simulink model "DroneControl"  (R2016a)
settings: Solver=VariableStepAuto  StartTime=0.0  StopTime=20  RelTol=1e-3
values from neighbouring files (symbols this model uses):
  SetPoint = 50    [DroneScript.m]
libraries: simulink x1
settings Model: Creator=Radu  LastModifiedBy=Radu

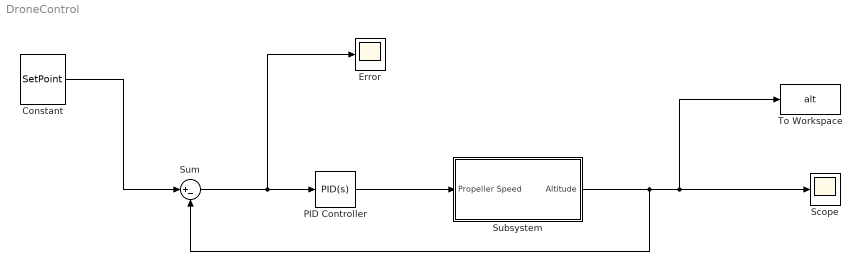
== system DroneControl ==
  Constant : Constant  Value=SetPoint
  "Error " : Scope
  PID Controller : simulink/Continuous/PID Controller  Controller=PID  TimeDomain=Continuous-time  SampleTime=-1  IntegratorMethod=Forward Euler  FilterMethod=Forward Euler  Form=Parallel  UseFilter=on  ControllerParametersSource=internal  P=10  I=1  D=0.1  N=100  InitialConditionSource=internal  InitialConditionForIntegrator=0  InitialConditionForFilter=0  ExternalReset=none  LimitOutput=off  UpperSaturationLimit=inf  LowerSaturationLimit=-inf  LinearizeAsGain=on  AntiWindupMode=none  Kb=1  TrackingMode=off  Kt=1  PParamMin=[]  PParamMax=[]  IParamMin=[]  IParamMax=[]  DParamMin=[]  DParamMax=[]  NParamMin=[]  NParamMax=[]  KbParamMin=[]  KbParamMax=[]  KtParamMin=[]  KtParamMax=[]  POutMin=[]  POutMax=[]  IOutMin=[]  IOutMax=[]  DOutMin=[]  DOutMax=[]  NOutMin=[]  NOutMax=[]  KbOutMin=[]  KbOutMax=[]  KtOutMin=[]  KtOutMax=[]  IntegratorOutMin=[]  IntegratorOutMax=[]  FilterOutMin=[]  FilterOutMax=[]  SumOutMin=[]  SumOutMax=[]  SumI1OutMin=[]  SumI1OutMax=[]  SumI2OutMin=[]  SumI2OutMax=[]  SumI3OutMin=[]  SumI3OutMax=[]  SumDOutMin=[]  SumDOutMax=[]  SaturationOutMin=[]  SaturationOutMax=[]  IntegratorContinuousStateAttributes=''  IntegratorStateMustResolveToSignalObject=off  IntegratorRTWStateStorageClass=Auto  FilterContinuousStateAttributes=''  FilterStateMustResolveToSignalObject=off  FilterRTWStateStorageClass=Auto  DifferentiatorICPrevScaledInput=0  DifferentiatorOutMin=[]  DifferentiatorOutMax=[]
  Scope : Scope
  Subsystem : Subsystem
  Sum : Sum  Inputs=|+-
  To Workspace : ToWorkspace  VariableName=alt  SaveFormat=Timeseries  SampleTime=-1
  wires:
  Subsystem/1(Altitude) -> To Workspace/1, Scope/1, Sum/2
  PID Controller/1 -> Subsystem/1(Propeller Speed)
  Sum/1 -> "Error "/1, PID Controller/1
  Constant/1 -> Sum/1

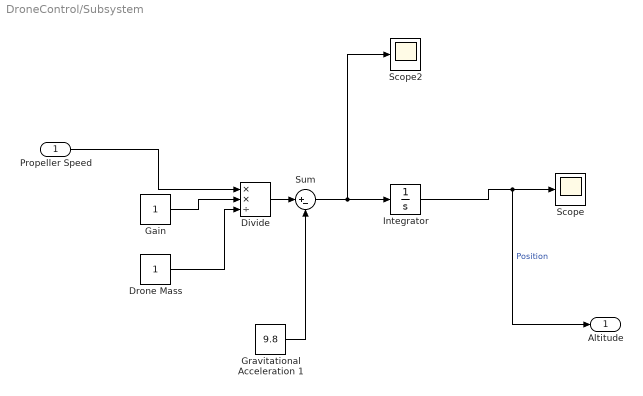
== system DroneControl/Subsystem ==
  Propeller Speed : Inport
  Divide : Product  Inputs=**/
  "Drone Mass " : Constant
  "Gain " : Constant
  Gravitational Acceleration 1 : Constant  Value=9.8
  Integrator : Integrator  LimitOutput=on  LowerSaturationLimit=0
  Scope : Scope
  Scope2 : Scope
  Sum : Sum  Inputs=|+-
  Altitude : Outport
  wires:
  Divide/1 -> Sum/1
  Gravitational Acceleration 1/1 -> Sum/2
  Integrator/1 -> Altitude/1, Scope/1  "Position"
  "Drone Mass "/1 -> Divide/3
  "Gain "/1 -> Divide/2
  Sum/1 -> Integrator/1, Scope2/1
  Propeller Speed/1 -> Divide/1
